simulink model "watermelon_simulink"  (R2017b)
settings: Solver=ode14x  StartTime=0.0  StopTime=10000  FixedStep=.1  RelTol=1e-3
settings Model: Creator=Harrison  LastModifiedBy=Harrison
settings DataIOCC: SaveFormat=Array

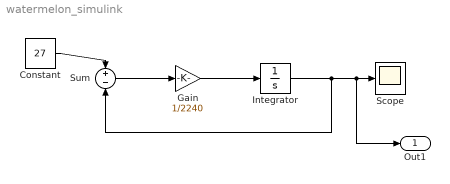
== system watermelon_simulink ==
  Constant : Constant  Value=27
  Gain : Gain  Gain=1/2240
  Integrator : Integrator  InitialCondition=5
  Scope : Scope
  Sum : Sum  Inputs=+-
  Out1 : Outport
  wires:
  Constant/1 -> Sum/1
  Sum/1 -> Gain/1
  Gain/1 -> Integrator/1
  Integrator/1 -> Sum/2, Out1/1, Scope/1
